simulink model "EvilSpagetty"  (R2020b)
settings: Solver=VariableStepAuto  StartTime=0.0  StopTime=3  RelTol=1e-3
(part 6 of 7)

== matlab function EvilSpagetty/Gt ==
  data: u1 input; y output; u2 input; u3 input; u4 input; u5 input
function y = fcn(u1,u2,u3,u4,u5)
theta1=u1;
theta2=u2;
theta3=u3;
theta4=u4;
theta5=u5;
Z=[                                                                                                                                                                                                                                                                                                                                                                                                                                                                                                                                                                                                                                                      0;
(3760780387158609*cos(theta2 + theta3 + theta4))/18014398509481984 + (5420822544825009913017827798490102737^(1/2)*cos(theta2 + theta3 + atan(2453075261925431/2328264703002381824)))/4611686018427387904 + (7528900944657674369452424878476848585^(1/2)*cos(theta2 - atan(1739956546642339/2743883728806468608)))/2305843009213693952 + (2207326208092009460722330602888339289^(1/2)*cos(theta2 + theta3 + theta4 + theta5 - atan(1485701483717825792/4160453179700955)))/73786976294838206464 - (2207326208092009460722330602888339289^(1/2)*cos(theta2 + theta3 + theta4 - theta5 + atan(1485701483717825792/4160453179700955)))/73786976294838206464;
                                                                                                                             (3760780387158609*cos(theta2 + theta3 + theta4))/18014398509481984 + (5420822544825009913017827798490102737^(1/2)*cos(theta2 + theta3 + atan(2453075261925431/2328264703002381824)))/4611686018427387904 + (2207326208092009460722330602888339289^(1/2)*cos(theta2 + theta3 + theta4 + theta5 - atan(1485701483717825792/4160453179700955)))/73786976294838206464 - (2207326208092009460722330602888339289^(1/2)*cos(theta2 + theta3 + theta4 - theta5 + atan(1485701483717825792/4160453179700955)))/73786976294838206464;
                                                                                                                                                                                                                                                                   (3760780387158609*cos(theta2 + theta3 + theta4))/18014398509481984 + (2207326208092009460722330602888339289^(1/2)*cos(theta2 + theta3 + theta4 + theta5 - atan(1485701483717825792/4160453179700955)))/73786976294838206464 - (2207326208092009460722330602888339289^(1/2)*cos(theta2 + theta3 + theta4 - theta5 + atan(1485701483717825792/4160453179700955)))/73786976294838206464;
                                                                                                                                                                                                                                                                                                                                                                                                         (2207326208092009460722330602888339289^(1/2)*(cos(theta2 + theta3 + theta4 + theta5 - atan(1485701483717825792/4160453179700955)) + cos(theta2 + theta3 + theta4 - theta5 + atan(1485701483717825792/4160453179700955))))/73786976294838206464];
y = Z;
